simulink model "Admittance"  (R2023b)
settings: Solver=VariableStepAuto  StartTime=0.0  StopTime=10.0  RelTol=1e-3
undefined symbols (not defined in the file or in its folder): D, K, M_inv
libraries: slpidlib x1, simulink x1
settings Model: Creator=sayeholoumi  LastModifiedBy=sayeholoumi

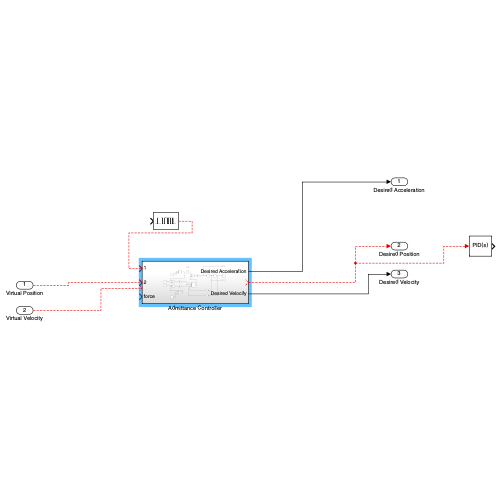
[thumbnail: Simulink's stored preview of the top-level diagram]
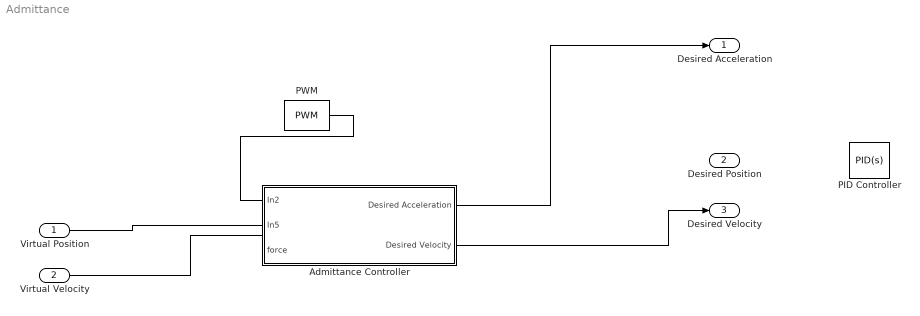
== system Admittance ==
  Virtual Position : Inport
  Virtual Velocity : Inport  Port=2
  Admittance Controller : Subsystem
  PID Controller : slpidlib/PID Controller  Controller=PID  Form=Parallel  TimeDomain=Continuous-time  UseExternalTs=off  SampleTime=-1  IntegratorMethod=Forward Euler  FilterMethod=Forward Euler  ControllerParametersSource=internal  P=1  I=0  UseKiTs=off  D=1  N=100  UseFilter=on  TunerSelectOption=Transfer Function Based (PID Tuner App)  InitialConditionSource=internal  InitialConditionForIntegrator=0  InitialConditionForFilter=0  DifferentiatorICPrevScaledInput=0  ExternalReset=none  TrackingMode=off  Kt=1  LimitOutput=off  SatLimitsSource=internal  UpperSaturationLimit=inf  LowerSaturationLimit=-inf  LinearizeAsGain=on  AntiWindupMode=none  Kb=1  LimitIntegrator=off  UpperIntegratorSaturationLimit=inf  LowerIntegratorSaturationLimit=-inf  POutMin=[]  POutMax=[]  IOutMin=[]  IOutMax=[]  DOutMin=[]  DOutMax=[]  NOutMin=[]  NOutMax=[]  SumOutMin=[]  SumOutMax=[]  SaturationOutMin=[]  SaturationOutMax=[]  PParamMin=[]  PParamMax=[]  IParamMin=[]  IParamMax=[]  DParamMin=[]  DParamMax=[]  NParamMin=[]  NParamMax=[]  KbParamMin=[]  KbParamMax=[]  KtParamMin=[]  KtParamMax=[]  KbOutMin=[]  KbOutMax=[]  KtOutMin=[]  KtOutMax=[]  IntegratorOutMin=[]  IntegratorOutMax=[]  FilterOutMin=[]  FilterOutMax=[]  SumI1OutMin=[]  SumI1OutMax=[]  SumI2OutMin=[]  SumI2OutMax=[]  SumI3OutMin=[]  SumI3OutMax=[]  SumI4OutMin=[]  SumI4OutMax=[]  SumDOutMin=[]  SumDOutMax=[]  DifferentiatorOutMin=[]  DifferentiatorOutMax=[]  FilterDiffOutCoefMin=[]  FilterDiffOutCoefMax=[]  ReciprocalOutMin=[]  ReciprocalOutMax=[]  SumDenOutMin=[]  SumDenOutMax=[]  SumNumOutMin=[]  SumNumOutMax=[]  DivideOutMin=[]  DivideOutMax=[]  UdiffTsProdOutMin=[]  UdiffTsProdOutMax=[]  NTsProdOutMin=[]  NTsProdOutMax=[]  UintegralTsProdOutMin=[]  UintegralTsProdOutMax=[]  UngainTsProdOutMin=[]  UngainTsProdOutMax=[]  ClampingZeroOutDataTypeStr=Inherit: Inherit via back propagation  ClampingZeroOutMin=[]  ClampingZeroOutMax=[]  FilterDenConstantOutDataTypeStr=Inherit: Inherit via back propagation  FilterDenConstantOutMin=[]  FilterDenConstantOutMax=[]  PCopyOutDataTypeStr=Inherit: Inherit via back propagation  PCopyOutMin=[]  PCopyOutMax=[]  NCopyOutDataTypeStr=Inherit: Inherit via back propagation  NCopyOutMin=[]  NCopyOutMax=[]  IntegratorContinuousStateAttributes=''  IntegratorStateMustResolveToSignalObject=off  IntegratorRTWStateStorageClass=Auto  FilterContinuousStateAttributes=''  FilterStateMustResolveToSignalObject=off  FilterRTWStateStorageClass=Auto  ParallelPVariant=InternalParameters  IdealPVariant=Disabled  IVariant=InternalParameters  DVariant=InternalParameters  IntegratorVariant=Continuous  SatVariant=Disabled  AWVariant=Passthrough  PCopyVariant=Disabled  TRVariant=Disabled  FdbkBlocksVariant=Forward  IdealPFdbkVariant=Disabled  SatFdbkVariant=Disabled  DerivativeFilterVariant=ContFilter  NVariant=InternalParameters  NCopyVariant=Disabled  FilterICVariant=InternalICsFilter  IntegratorICVariant=InternalICs  ExternalResetVariant=Disabled  TRSumVariant=Passthrough  SumFdbkVariant=Disabled  SumVariant=Sum_PID  TsampFilterVariant=InternalTs  TsampNgainVariant=Passthrough  TsampIntegralVariant=Disabled_SignalSpec  ExternalSaturationOutDataTypeStr=Inherit: Same as second input
  PWM : simulink/Discontinuities/PWM  DisableCoverage=on  Period=1  InitialDelay=0  DisallowZeroDutyCycle=off  RunAtFixedTimeIntervals=off  SampleTime=0.1
  Desired Acceleration : Outport
  Desired Position : Outport  Port=2
  Desired Velocity : Outport  Port=3
  wires:
  PWM/1 -> ?
  Virtual Position/1 -> ?
  Virtual Velocity/1 -> ?
  Admittance Controller/1(Desired Acceleration) -> Desired Acceleration/1
  ? -> Desired Position/1, PID Controller/1
  Admittance Controller/2(Desired Velocity) -> Desired Velocity/1

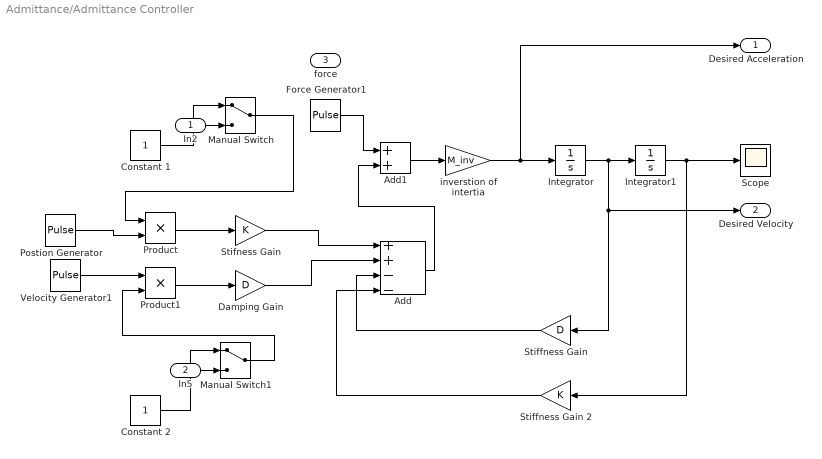
== system Admittance/Admittance Controller ==
  In2 : Inport
  In5 : Inport  Port=2
  force : Inport  Port=3
  Add : Sum  Inputs=++--
  Add1 : Sum
  Constant 1 : Constant
  Constant 2 : Constant
  Damping Gain : Gain  Gain=D
  Force Generator1 : DiscretePulseGenerator  PulseType=Time based  Period=10  PulseWidth=5
  Integrator : Integrator
  Integrator1 : Integrator
  Manual Switch : ManualSwitch
  Manual Switch1 : ManualSwitch
  Postion Generator : DiscretePulseGenerator  PulseType=Time based  Period=10  PulseWidth=5
  Product : Product
  Product1 : Product
  Scope : Scope
  Stiffness Gain : Gain  Gain=D
  Stiffness Gain 2 : Gain  Gain=K
  Stifness Gain : Gain  Gain=K
  Velocity Generator1 : DiscretePulseGenerator  PulseType=Time based  Period=10  PulseWidth=5
  inverstion of intertia : Gain  Gain=M_inv
  Desired Acceleration : Outport
  Desired Velocity : Outport  Port=2
  wires:
  In2/1 -> Manual Switch/2
  In5/1 -> Manual Switch1/2
  Product/1 -> Stifness Gain/1
  Damping Gain/1 -> Add/2
  Add/1 -> Add1/2
  Manual Switch1/1 -> Product1/2
  Add1/1 -> inverstion of intertia/1
  Velocity Generator1/1 -> Product1/1
  Manual Switch/1 -> Product/1
  Stiffness Gain/1 -> Add/3
  inverstion of intertia/1 -> Desired Acceleration/1, Integrator/1
  Constant 2/1 -> Manual Switch1/1
  Stiffness Gain 2/1 -> Add/4
  Integrator1/1 -> Scope/1, Stiffness Gain 2/1
  Constant 1/1 -> Manual Switch/1
  Postion Generator/1 -> Product/2
  Stifness Gain/1 -> Add/1
  Force Generator1/1 -> Add1/1
  Integrator/1 -> Desired Velocity/1, Stiffness Gain/1, Integrator1/1
  Product1/1 -> Damping Gain/1
